simulink model "sampleModel548_pp_1566_1"  (R2021a)
settings: Solver=VariableStepAuto  StartTime=0.0  StopTime=10.0  RelTol=1e-3
undefined symbols (not defined in the file or in its folder): DiscIntNeverNeededParam, Newton, Raphson
libraries: simulink x54, pid_lib x8
(part 1 of 2)
settings Model: Creator=user  LastModifiedBy=user

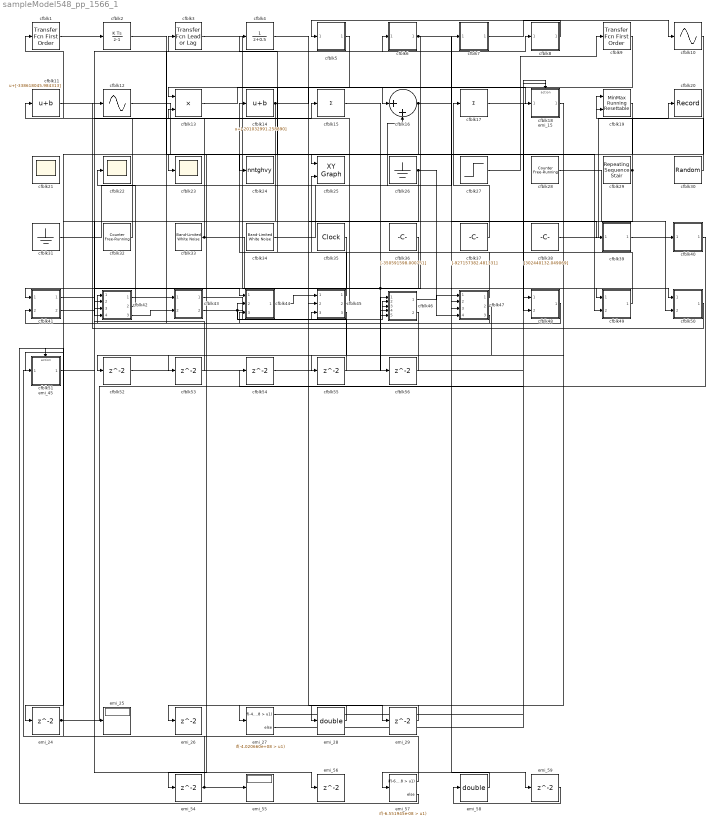
== system sampleModel548_pp_1566_1 ==
  cfblk1 : simulink/Discrete/Transfer Fcn First Order  PoleZ=0.95  ICPrevOutput=0.0  DoSatur=off
  cfblk10 : Sin  TimeSource=Use external signal  SampleTime=0
  cfblk11 : Bias  Bias=[-338618045.984313]
  cfblk12 : Sin  TimeSource=Use external signal  SampleTime=0
  cfblk13 : Product
  cfblk14 : Bias  Bias=[-201032991.258890]
  cfblk15 : Sum  Inputs=+
  cfblk16 : Sum  Inputs=|++
  cfblk17 : Sum  Inputs=+
  cfblk18 : Subsystem  TreatAsAtomicUnit=on
  cfblk19 : simulink/Math Operations/MinMax Running Resettable  Function=min  vinit=0.0
  cfblk2 : DiscreteIntegrator  ICPrevOutput=DiscIntNeverNeededParam  ICPrevScaledInput=DiscIntNeverNeededParam
  cfblk20 : Record  FileSettingsInternal="{\"entries\":[{\"content\":{\"excelSettings\":{\"content\":{},\"type\":\"Streamout.ExcelSettings\"}},\"type\":\"Streamout.FileSettingStorage\",\"uuid\":\"7a93cd99-5695-4368-9288-ae4d8ae2b655\"}],\"packageUris\":[\"http://schema.mathworks.com/mf0/streamout_blocks/R2020a\"],\"version\":\"1.0\"}"  SignalsInternal="{\"entries\":[{\"content\":{\"signals\":[{\"content\":{\"blockPath\":[\"sampleModel548_pp_1566_1/cfblk20\"],\"channel\":[],\"dimensions\":[1],\"domain\":\"samplemodel548_pp_1566_1/cfblk20\",\"lineColor\":\"#b746ff\",\"plots\":[1],\"port\":1,\"sid\":[\"\"],\"signalID\":1494751,\"signalName\":\"cfblk38\"},\"type\":\"RecordBlkView.Signal\",\"uuid\":\"c7f9f908-5acf-44de-b635-a9ae11b3c0ae\"}]},\"type\":\"RecordBlkView.InputSignals\",\"uuid\":\"681cfd0e-31b9-4ca3-9765-5b08f12cf705\"}],\"packageUris\":[\"http://schema.mathworks.com/mf0/streamout_blocks/R2020a\"],\"version\":\"1.0\"}"  VisualizationBindings="{\"sparklinesplugin\":{\"info\":[{\"bindingParametersList\":[],\"subplotID\":1}]}}"
  cfblk21 : Scope
      settings: Floating=on
  cfblk22 : Scope
  cfblk23 : Scope
  cfblk24 : ToWorkspace  VariableName=nntghvy  SaveFormat=Timeseries  SampleTime=-1
  cfblk25 : simulink/Sinks/XY Graph  xmin=-1  xmax=1  ymin=-1  ymax=1  st=-1
  cfblk26 : Ground
  cfblk27 : Step  Time=[40.000000]  Before=[709789414.662240]  After=[776735056.730233]  SampleTime=0
  cfblk28 : simulink/Sources/Counter Free-Running  NumBits=[29.000000]  tsamp=-1
  cfblk29 : simulink/Sources/Repeating Sequence Stair  OutValues=[661742616.793887, -192762915.667570]  tsamp=-1  OutMin=[]  OutMax=[]  OutDataTypeStr=double  OutputDataTypeScalingMode=double  OutDataType=fixdt(0,8)  ConRadixGroup=Best Precision: Vector-wise  OutScaling=2^-12
  cfblk3 : simulink/Discrete/Transfer Fcn Lead or Lag  PoleZ=0.95  ZeroZ=0.75  ICPrevOutput=0.0  ICPrevInput=0.0  DoSatur=off
      settings: SourceProductBaseCode=SL
  cfblk30 : UniformRandomNumber  Minimum=[-3848918818.431031]  Maximum=[6546494102.083925]  Seed=[18894411.000000]  SampleTime=0.1
  cfblk31 : Ground
  cfblk32 : simulink/Sources/Counter Free-Running  NumBits=[47.000000]  tsamp=-1
  cfblk33 : simulink/Sources/Band-Limited White Noise  Cov=[521319541.609249]  Ts=0.1  seed=[6000899315.000000]
  cfblk34 : simulink/Sources/Band-Limited White Noise  Cov=[5907275539.818776]  Ts=0.1  seed=[7621611147.000000]
  cfblk35 : DigitalClock
  cfblk36 : Constant  Value=[-350591598.000751]  SampleTime=1
  cfblk37 : Constant  Value=[-927157382.481331]  SampleTime=1
  cfblk38 : Constant  Value=[302440132.049069]  SampleTime=1
  cfblk39 : Subsystem  TreatAsAtomicUnit=on
  cfblk4 : DiscreteTransferFcn  SampleTime=1
  cfblk40 : Subsystem
  cfblk41 : Subsystem
  cfblk42 : Subsystem
  cfblk43 : Subsystem
  cfblk44 : Subsystem
  cfblk45 : Subsystem
  cfblk46 : Subsystem
  cfblk47 : Subsystem
  cfblk48 : Subsystem
  cfblk49 : Subsystem
  cfblk5 : Subsystem  TreatAsAtomicUnit=on
  cfblk50 : Subsystem
  cfblk51 : Subsystem  TreatAsAtomicUnit=on
  cfblk{52..56} (5 alike) : Delay  SampleTime=1
  cfblk6 : Subsystem  TreatAsAtomicUnit=on
  cfblk7 : Subsystem  TreatAsAtomicUnit=on
  cfblk8 : Subsystem  TreatAsAtomicUnit=on
  cfblk9 : simulink/Discrete/Transfer Fcn First Order  PoleZ=0.95  ICPrevOutput=0.0  DoSatur=off
  emi_15 : Subsystem  TreatAsAtomicUnit=on
  emi_24 : Delay
  emi_25 : Display
  emi_26 : Delay
  emi_27 : If  IfExpression=-4.020660e+08 > u1
  emi_28 : DataTypeConversion  OutDataTypeStr=double
  emi_29 : Delay  InitialCondition=-201032991.2589
  emi_45 : Subsystem  TreatAsAtomicUnit=on
  emi_54 : Delay  SampleTime=1
  emi_55 : Display
  emi_56 : Delay  SampleTime=1
  emi_57 : If  IfExpression=-6.551945e-08 > u1  SampleTime=1
  emi_58 : DataTypeConversion  OutDataTypeStr=double
  emi_59 : Delay  InitialCondition=-3.276e-08
  wires:
  cfblk48/1(cfblk2) -> cfblk42/1(cfblk1)
  cfblk50/1(cfblk2) -> cfblk12/1
  cfblk27/1 -> cfblk9/1
  cfblk3/1 -> cfblk48/2(cfblk11)
  cfblk47/1(cfblk2) -> cfblk14/1
  cfblk9/1 -> cfblk24/1
  cfblk33/1 -> cfblk47/2(cfblk13), cfblk46/5(cfblk16), cfblk11/1
  cfblk13/1 -> cfblk16/1
  cfblk2/1 -> cfblk25/1
  cfblk42/2(cfblk15) -> cfblk22/1
  cfblk1/1 -> cfblk2/1
  cfblk45/1(cfblk2) -> cfblk4/1
  cfblk29/1 -> cfblk19/1, cfblk47/3(cfblk14)
  cfblk36/1 -> cfblk41/1(cfblk1)
  cfblk10/1 -> cfblk23/1
  cfblk31/1 -> cfblk16/2
  cfblk26/1 -> cfblk42/2(cfblk12), cfblk47/4(cfblk15)
  cfblk49/1(cfblk2) -> cfblk25/2
  cfblk41/1(cfblk2) -> cfblk15/1
  cfblk32/1 -> cfblk1/1
  cfblk37/1 -> cfblk17/1
  cfblk30/1 -> cfblk19/2
  cfblk17/1 -> cfblk50/1(cfblk1)
  cfblk28/1 -> cfblk50/2(cfblk7)
  cfblk12/1 -> cfblk49/2(cfblk8)
  cfblk38/1 -> cfblk20/1
  cfblk43/1(cfblk2) -> cfblk46/2(cfblk13)
  cfblk44/1(cfblk2) -> cfblk45/1(cfblk1)
  cfblk43/2(cfblk14) -> cfblk46/3(cfblk14), cfblk45/3(cfblk15)
  cfblk19/1 -> cfblk46/4(cfblk15)
  cfblk41/2(cfblk11) -> cfblk44/1(cfblk1)
  cfblk46/1(cfblk2) -> cfblk47/1(cfblk1)
  cfblk45/2(cfblk16) -> cfblk13/2
  cfblk46/2(cfblk17) -> cfblk41/2(cfblk10)
  cfblk35/1 -> cfblk42/4(cfblk14)
  cfblk42/3(cfblk16) -> cfblk43/2(cfblk13)
  cfblk47/3(cfblk17) -> cfblk44/3(cfblk11)
  cfblk52/1 -> cfblk48/1(cfblk1)
  cfblk47/2(cfblk16) -> cfblk53/1
  cfblk53/1 -> cfblk42/3(cfblk13)
  cfblk40/1(cfblk2) -> cfblk54/1
  cfblk54/1 -> cfblk46/1(cfblk1)
  cfblk45/3(cfblk17) -> cfblk55/1
  cfblk55/1 -> cfblk44/2(cfblk10)
  cfblk15/1 -> cfblk56/1
  cfblk56/1 -> cfblk43/1(cfblk1)
  cfblk4/1 -> cfblk39/1(emi_10)
  cfblk39/1(emi_11) -> cfblk40/1(cfblk1)
  cfblk14/1 -> cfblk18/1(emi_13), emi_24/1, emi_29/1
  cfblk18/1(emi_14) -> cfblk52/1
  emi_24/1 -> emi_15/1(emi_22), emi_25/1
  emi_15/1(emi_23) -> emi_26/1
  emi_27/2 -> cfblk18/Action
  emi_27/1 -> emi_15/Action
  emi_28/1 -> emi_27/1
  emi_29/1 -> emi_28/1
  cfblk5/1(emi_32) -> cfblk13/1
  cfblk11/1 -> cfblk6/1(emi_34)
  cfblk6/1(emi_35) -> cfblk45/2(cfblk14), cfblk49/1(cfblk1)
  cfblk34/1 -> cfblk7/1(emi_37)
  cfblk7/1(emi_38) -> cfblk10/1
  cfblk42/1(cfblk2) -> cfblk8/1(emi_40)
  cfblk8/1(emi_41) -> cfblk5/1(emi_31)
  cfblk16/1 -> cfblk51/1(emi_43), emi_54/1, emi_59/1
  cfblk51/1(emi_44) -> cfblk3/1
  emi_54/1 -> emi_45/1(emi_52), emi_55/1
  emi_45/1(emi_53) -> emi_56/1
  emi_57/2 -> cfblk51/Action
  emi_57/1 -> emi_45/Action
  emi_58/1 -> emi_57/1
  emi_59/1 -> emi_58/1

== system sampleModel548_pp_1566_1/cfblk18 ==
  emi_13 : Inport
  Action Port : ActionPort  ActionPortLabel=else
  cfblk18 : Subsystem  TreatAsAtomicUnit=on
  emi_14 : Outport
  wires:
  emi_13/1 -> cfblk18/1(emi_7)
  cfblk18/1(emi_8) -> emi_14/1

== system sampleModel548_pp_1566_1/cfblk39 ==
  emi_10 : Inport  Partition=on  PartitionDimension=1  PartitionWidth=1  PartitionOffset=0
  For Each : ForEach  DisableCoverage=on
  cfblk39 : Subsystem
  emi_11 : Outport  ConcatenationDimension=1
  wires:
  emi_10/1 -> cfblk39/1(cfblk1)
  cfblk39/1(cfblk2) -> emi_11/1

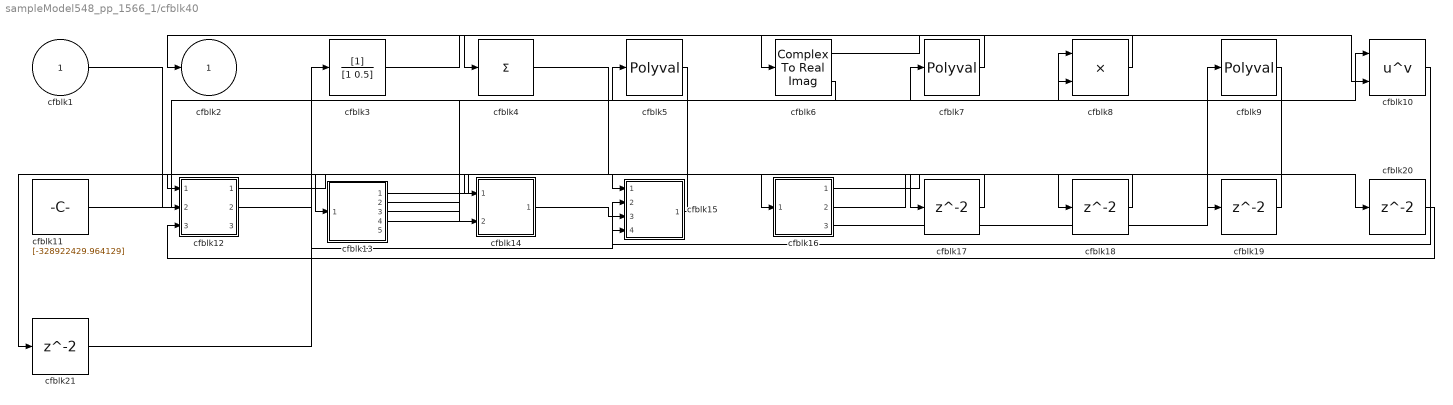
== system sampleModel548_pp_1566_1/cfblk40 ==
  cfblk1 : Inport
  cfblk10 : Math  Operator=pow  SaturateOnIntegerOverflow=on
  cfblk11 : Constant  Value=[-328922429.964129]  SampleTime=1
  cfblk12 : Subsystem
  cfblk13 : Subsystem
  cfblk14 : Subsystem
  cfblk15 : Subsystem
  cfblk16 : Subsystem
  cfblk{17..21} (5 alike) : Delay  SampleTime=1
  cfblk3 : DiscreteFilter  SampleTime=1
  cfblk4 : Sum  Inputs=+
  cfblk5 : Polyval  Coefs=[ +2.081618890e-019, -1.441693666e-014, +4.719686976e-010, -8.536869453e-006, +1.621573104e-001, -8.087801117e+001 ]
  cfblk6 : ComplexToRealImag
  cfblk7 : Polyval  Coefs=[ +2.081618890e-019, -1.441693666e-014, +4.719686976e-010, -8.536869453e-006, +1.621573104e-001, -8.087801117e+001 ]
  cfblk8 : Product
  cfblk9 : Polyval  Coefs=[ +2.081618890e-019, -1.441693666e-014, +4.719686976e-010, -8.536869453e-006, +1.621573104e-001, -8.087801117e+001 ]
  cfblk2 : Outport
  wires:
  cfblk7/1 -> cfblk4/1
  cfblk11/1 -> cfblk10/1
  cfblk3/1 -> cfblk6/1
  cfblk10/1 -> cfblk15/2(cfblk7)
  cfblk6/1 -> cfblk10/2
  cfblk8/1 -> cfblk2/1
  cfblk6/2 -> cfblk5/1
  cfblk12/1(cfblk2) -> cfblk16/1(cfblk1)
  cfblk5/1 -> cfblk12/2(cfblk11)
  cfblk13/2(cfblk14) -> cfblk7/1
  cfblk1/1 -> cfblk14/2(cfblk9)
  cfblk14/1(cfblk2) -> cfblk15/3(cfblk8)
  cfblk16/3(cfblk16) -> cfblk9/1
  cfblk15/1(cfblk2) -> cfblk13/1(cfblk1)
  cfblk13/3(cfblk15) -> cfblk8/1
  cfblk13/4(cfblk16) -> cfblk8/2
  cfblk12/2(cfblk13) -> cfblk15/4(cfblk9)
  cfblk13/1(cfblk2) -> cfblk17/1
  cfblk17/1 -> cfblk14/1(cfblk1)
  cfblk4/1 -> cfblk18/1
  cfblk18/1 -> cfblk15/1(cfblk1)
  cfblk16/1(cfblk2) -> cfblk19/1
  cfblk19/1 -> cfblk12/1(cfblk1)
  cfblk16/2(cfblk15) -> cfblk20/1
  cfblk20/1 -> cfblk12/3(cfblk12)
  cfblk9/1 -> cfblk21/1
  cfblk21/1 -> cfblk3/1

== system sampleModel548_pp_1566_1/cfblk41 ==
  cfblk1 : Inport
  cfblk10 : Inport  Port=2
  cfblk3 : Delay  ShowEnablePort=on  SampleTime=1
      settings: InputPortMap=u0,e6
  cfblk4 : Product  Inputs=*
  cfblk5 : Sqrt  SaturateOnIntegerOverflow=on
  cfblk6 : Sin  TimeSource=Use external signal  SampleTime=0
  cfblk7 : Subsystem
  cfblk8 : Subsystem
  cfblk9 : Subsystem
  cfblk2 : Outport
  cfblk11 : Outport  Port=2
  wires:
  cfblk6/1 -> cfblk2/1
  cfblk3/1 -> cfblk6/1
  cfblk10/1 -> cfblk3/1
  cfblk1/1 -> cfblk7/1(cfblk1)
  cfblk8/1(cfblk2) -> cfblk4/1
  cfblk8/2(cfblk10) -> cfblk5/1
  cfblk5/1 -> cfblk11/1
  cfblk9/1(cfblk2) -> cfblk3/2
  cfblk9/2(cfblk15) -> cfblk8/1(cfblk1)
  cfblk7/1(cfblk2) -> cfblk9/1(cfblk1)
  cfblk7/2(cfblk7) -> cfblk9/2(cfblk13)
  cfblk7/3(cfblk8) -> cfblk9/3(cfblk14)

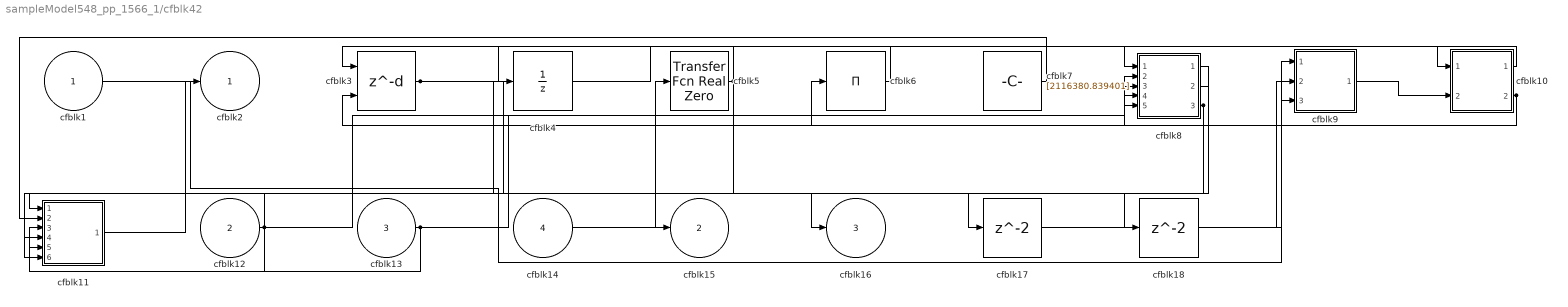
== system sampleModel548_pp_1566_1/cfblk42 ==
  cfblk1 : Inport
  cfblk12 : Inport  Port=2
  cfblk13 : Inport  Port=3
  cfblk14 : Inport  Port=4
  cfblk10 : Subsystem
  cfblk11 : Subsystem
  cfblk17 : Delay  SampleTime=1
  cfblk18 : Delay  SampleTime=1
  cfblk3 : Delay  DelayLengthSource=Input port  SampleTime=1
      settings: InputPortMap=u0,p1
  cfblk4 : UnitDelay  HasFrameUpgradeWarning=on
  cfblk5 : simulink/Discrete/Transfer Fcn Real Zero  ZeroZ=0.75  ICPrevInput=0.0  DoSatur=off
      settings: SourceProductBaseCode=SL
  cfblk6 : Product  Inputs=*
  cfblk7 : Constant  Value=[2116380.839401]  SampleTime=1
  cfblk8 : Subsystem
  cfblk9 : Subsystem
  cfblk2 : Outport
  cfblk15 : Outport  Port=2
  cfblk16 : Outport  Port=3
  wires:
  cfblk3/1 -> cfblk16/1, cfblk18/1
  cfblk6/1 -> cfblk3/1
  cfblk14/1 -> cfblk5/1
  cfblk12/1 -> cfblk11/1(cfblk1), cfblk11/5(cfblk15), cfblk8/4(cfblk13)
  cfblk5/1 -> cfblk4/1, cfblk11/6(cfblk16)
  cfblk7/1 -> cfblk11/2(cfblk12)
  cfblk13/1 -> cfblk11/3(cfblk13), cfblk8/3(cfblk12)
  cfblk1/1 -> cfblk9/1(cfblk1)
  cfblk4/1 -> cfblk10/1(cfblk1)
  cfblk10/1(cfblk2) -> cfblk8/1(cfblk1)
  cfblk9/1(cfblk2) -> cfblk10/2(cfblk16)
  cfblk11/1(cfblk2) -> cfblk2/1
  cfblk10/2(cfblk17) -> cfblk6/1, cfblk8/2(cfblk11), cfblk8/5(cfblk14)
  cfblk8/1(cfblk2) -> cfblk15/1
  cfblk8/3(cfblk16) -> cfblk11/4(cfblk14), cfblk3/2
  cfblk8/2(cfblk15) -> cfblk17/1
  cfblk17/1 -> cfblk9/2(cfblk6)
  cfblk18/1 -> cfblk9/3(cfblk7)

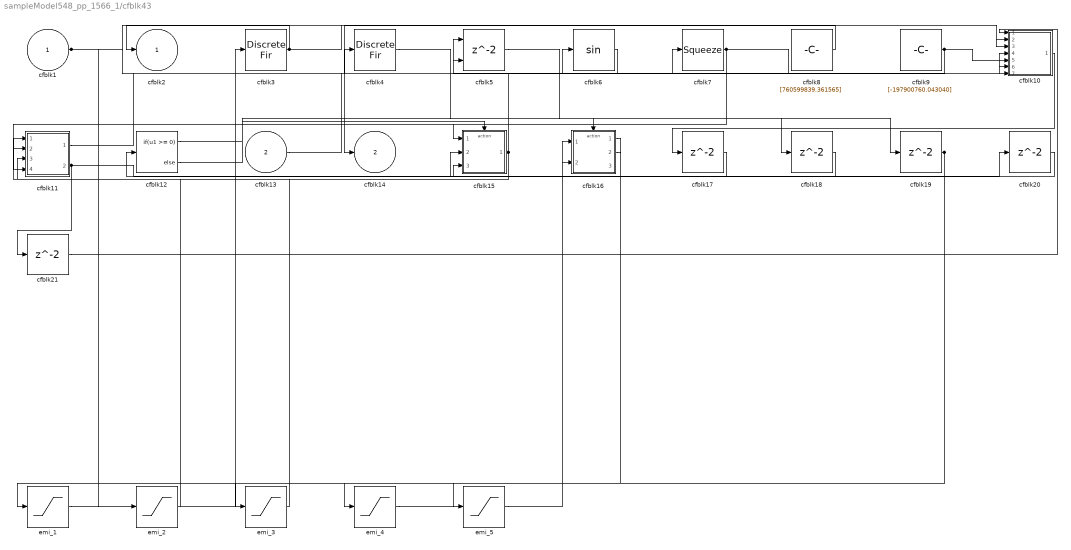
== system sampleModel548_pp_1566_1/cfblk43 ==
  cfblk1 : Inport
  cfblk13 : Inport  Port=2
  cfblk10 : Subsystem
  cfblk11 : Subsystem
  cfblk12 : If  IfExpression=u1 >= 0  SampleTime=1
  cfblk15 : Subsystem  TreatAsAtomicUnit=on
  cfblk16 : Subsystem  TreatAsAtomicUnit=on
  cfblk{17..21} (5 alike) : Delay  SampleTime=1
  cfblk3 : DiscreteFir  SampleTime=1
  cfblk4 : DiscreteFir  SampleTime=1
  cfblk5 : Delay  ShowEnablePort=on  SampleTime=1
      settings: InputPortMap=u0,e6
  cfblk6 : Trigonometry
  cfblk7 : Squeeze
  cfblk8 : Constant  Value=[760599839.361565]  SampleTime=1
  cfblk9 : Constant  Value=[-197900760.043040]  SampleTime=1
  emi_{1..5} (5 alike) : Saturate  UpperLimit=0  LowerLimit=0  ZeroCross=off
  cfblk2 : Outport
  cfblk14 : Outport  Port=2
  wires:
  cfblk15/1(cfblk2) -> cfblk5/1, cfblk11/3(cfblk15)
  cfblk8/1 -> cfblk14/1
  cfblk9/1 -> cfblk6/1, cfblk10/5(cfblk10)
  cfblk11/1(cfblk2) -> cfblk4/1
  cfblk6/1 -> cfblk5/2
  cfblk13/1 -> cfblk7/1
  cfblk11/2(cfblk17) -> cfblk20/1, cfblk21/1
  cfblk3/1 -> cfblk2/1, cfblk10/3(cfblk8)
  cfblk7/1 -> cfblk15/1(cfblk1), cfblk11/4(cfblk16), cfblk10/4(cfblk9), cfblk10/6(cfblk11)
  cfblk1/1 -> cfblk10/2(cfblk7), cfblk10/7(cfblk12), emi_2/1
  cfblk12/1 -> cfblk15/Action
  cfblk12/2 -> cfblk16/Action
  cfblk10/1(cfblk2) -> cfblk17/1
  cfblk17/1 -> cfblk15/2(cfblk10)
  cfblk5/1 -> cfblk18/1
  cfblk18/1 -> cfblk15/3(cfblk11)
  cfblk4/1 -> cfblk19/1
  cfblk20/1 -> cfblk12/1
  cfblk21/1 -> cfblk10/1(cfblk1)
  emi_1/1 -> cfblk3/1
  cfblk19/1 -> emi_1/1, emi_3/1
  emi_2/1 -> cfblk11/1(cfblk1)
  emi_3/1 -> cfblk11/2(cfblk14)
  emi_4/1 -> cfblk16/1(cfblk1)
  cfblk16/1(cfblk2) -> emi_4/1
  emi_5/1 -> cfblk16/2(cfblk9)
  cfblk16/2(cfblk10) -> emi_5/1

== system sampleModel548_pp_1566_1/cfblk44 ==
  cfblk1 : Inport
  cfblk10 : Inport  Port=2
  cfblk11 : Inport  Port=3
  cfblk3 : DiscreteFir  SampleTime=1
  cfblk4 : Delay  ShowEnablePort=on  SampleTime=1
      settings: InputPortMap=u0,e6
  cfblk5 : DiscreteStateSpace
  cfblk6 : Signum
  cfblk7 : Constant  Value=[-388627596.209569]  SampleTime=1
  cfblk8 : Constant  Value=[-19012046.520637]  SampleTime=1
  cfblk9 : Subsystem
  cfblk2 : Outport
  wires:
  cfblk8/1 -> cfblk5/1
  cfblk9/1(cfblk2) -> cfblk4/1
  cfblk1/1 -> cfblk4/2
  cfblk10/1 -> cfblk6/1
  cfblk5/1 -> cfblk3/1
  cfblk7/1 -> cfblk2/1
  cfblk3/1 -> cfblk9/1(cfblk1)
  cfblk6/1 -> cfblk9/2(cfblk11)

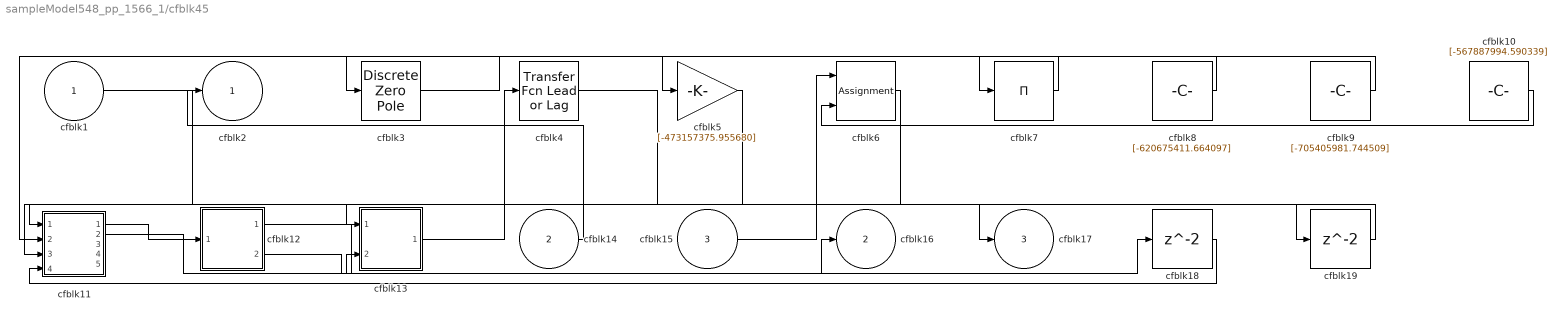
== system sampleModel548_pp_1566_1/cfblk45 ==
  cfblk1 : Inport
  cfblk14 : Inport  Port=2
  cfblk15 : Inport  Port=3
  cfblk10 : Constant  Value=[-567887994.590339]  SampleTime=1
  cfblk11 : Subsystem
  cfblk12 : Subsystem
  cfblk13 : Subsystem
  cfblk18 : Delay  SampleTime=1
  cfblk19 : Delay  SampleTime=1
  cfblk3 : DiscreteZeroPole  Poles=[0 0.5]  Gain=1
  cfblk4 : simulink/Discrete/Transfer Fcn Lead or Lag  PoleZ=0.95  ZeroZ=0.75  ICPrevOutput=0.0  ICPrevInput=0.0  DoSatur=off
      settings: SourceProductBaseCode=SL
  cfblk5 : Gain  Gain=[-473157375.955680]
  cfblk6 : Assignment  DiagnosticForDimensions=Warning  IndexOptions=Index vector (dialog)  Indices=1  OutputSizes=1
  cfblk7 : Product  Inputs=*
  cfblk8 : Constant  Value=[-620675411.664097]  SampleTime=1
  cfblk9 : Constant  Value=[-705405981.744509]  SampleTime=1
  cfblk2 : Outport
  cfblk16 : Outport  Port=2
  cfblk17 : Outport  Port=3
  wires:
  cfblk5/1 -> cfblk11/1(cfblk1)
  cfblk7/1 -> cfblk11/2(cfblk9)
  cfblk12/1(cfblk2) -> cfblk16/1
  cfblk1/1 -> cfblk17/1
  cfblk13/1(cfblk2) -> cfblk4/1
  cfblk3/1 -> cfblk7/1
  cfblk15/1 -> cfblk6/1
  cfblk9/1 -> cfblk3/1
  cfblk6/1 -> cfblk11/3(cfblk10)
  cfblk8/1 -> cfblk5/1
  cfblk11/1(cfblk2) -> cfblk12/1(cfblk1)
  cfblk10/1 -> cfblk6/2
  cfblk14/1 -> cfblk2/1
  cfblk11/2(cfblk12) -> cfblk13/2(cfblk9)
  cfblk12/2(cfblk10) -> cfblk18/1
  cfblk18/1 -> cfblk11/4(cfblk11)
  cfblk4/1 -> cfblk19/1
  cfblk19/1 -> cfblk13/1(cfblk1)

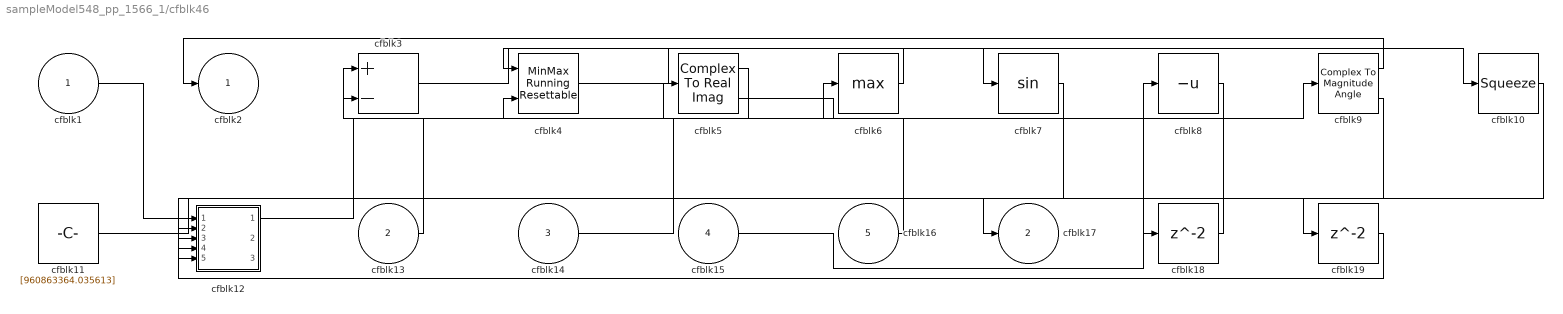
== system sampleModel548_pp_1566_1/cfblk46 ==
  cfblk1 : Inport
  cfblk13 : Inport  Port=2
  cfblk14 : Inport  Port=3
  cfblk15 : Inport  Port=4
  cfblk16 : Inport  Port=5
  cfblk10 : Squeeze
  cfblk11 : Constant  Value=[960863364.035613]  SampleTime=1
  cfblk12 : Subsystem
  cfblk18 : Delay  SampleTime=1
  cfblk19 : Delay  SampleTime=1
  cfblk3 : Sum  Inputs=+-
  cfblk4 : simulink/Math Operations/MinMax Running Resettable  Function=min  vinit=0.0
  cfblk5 : ComplexToRealImag
  cfblk6 : MinMax  Function=max
  cfblk7 : Trigonometry
  cfblk8 : UnaryMinus
  cfblk9 : ComplexToMagnitudeAngle
  cfblk2 : Outport
  cfblk17 : Outport  Port=2
  wires:
  cfblk3/1 -> cfblk7/1
  cfblk11/1 -> cfblk17/1
  cfblk9/1 -> cfblk2/1
  cfblk1/1 -> cfblk12/1(cfblk1)
  cfblk6/1 -> cfblk4/1
  cfblk13/1 -> cfblk3/1
  cfblk5/1 -> cfblk4/2
  cfblk4/1 -> cfblk10/1
  cfblk15/1 -> cfblk8/1
  cfblk7/1 -> cfblk12/2(cfblk11)
  cfblk16/1 -> cfblk3/2
  cfblk12/1(cfblk2) -> cfblk5/1
  cfblk5/2 -> cfblk9/1
  cfblk14/1 -> cfblk6/1
  cfblk8/1 -> cfblk12/5(cfblk14)
  cfblk10/1 -> cfblk18/1
  cfblk18/1 -> cfblk12/3(cfblk12)
  cfblk9/2 -> cfblk19/1
  cfblk19/1 -> cfblk12/4(cfblk13)

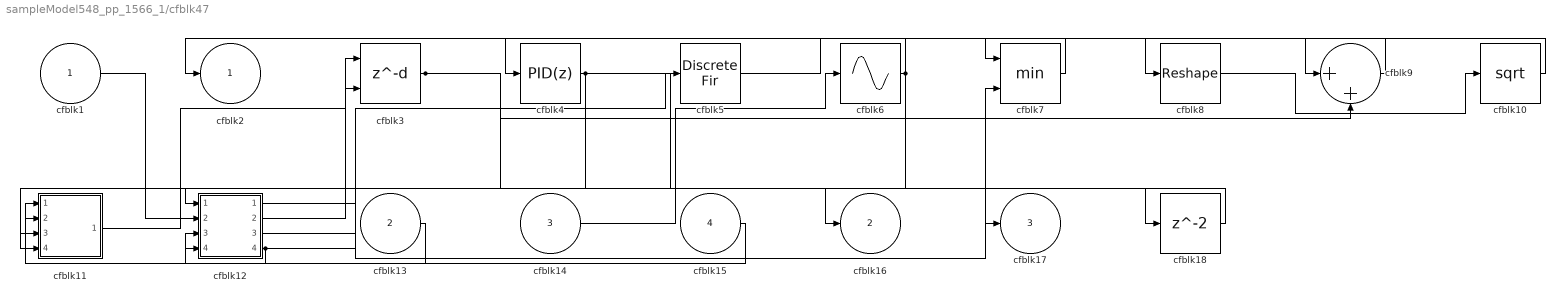
== system sampleModel548_pp_1566_1/cfblk47 ==
  cfblk1 : Inport
  cfblk13 : Inport  Port=2
  cfblk14 : Inport  Port=3
  cfblk15 : Inport  Port=4
  cfblk10 : Sqrt  SaturateOnIntegerOverflow=on
  cfblk11 : Subsystem
  cfblk12 : Subsystem
  cfblk18 : Delay  SampleTime=1
  cfblk3 : Delay  DelayLengthSource=Input port  SampleTime=1
      settings: InputPortMap=u0,p1
  cfblk4 : pid_lib/PID Controller  Controller=PID  Form=Parallel  TimeDomain=Discrete-time  UseExternalTs=off  SampleTime=1  IntegratorMethod=Forward Euler  FilterMethod=Forward Euler  ControllerParametersSource=internal  P=1  I=1  D=0  UseFilter=on  N=100  TunerSelectOption=Transfer Function Based (PID Tuner App)  InitialConditionSource=internal  InitialConditionForIntegrator=0  InitialConditionForFilter=0  DifferentiatorICPrevScaledInput=0  ExternalReset=none  TrackingMode=off  Kt=1  LimitOutput=off  SatLimitsSource=internal  UpperSaturationLimit=inf  LowerSaturationLimit=-inf  LinearizeAsGain=off  AntiWindupMode=none  Kb=1  POutMin=[]  POutMax=[]  IOutMin=[]  IOutMax=[]  DOutMin=[]  DOutMax=[]  NOutMin=[]  NOutMax=[]  SumOutMin=[]  SumOutMax=[]  SaturationOutMin=[]  SaturationOutMax=[]  PParamMin=[]  PParamMax=[]  IParamMin=[]  IParamMax=[]  DParamMin=[]  DParamMax=[]  NParamMin=[]  NParamMax=[]  KbParamMin=[]  KbParamMax=[]  KtParamMin=[]  KtParamMax=[]  KbOutMin=[]  KbOutMax=[]  KtOutMin=[]  KtOutMax=[]  IntegratorOutMin=[]  IntegratorOutMax=[]  FilterOutMin=[]  FilterOutMax=[]  SumI1OutMin=[]  SumI1OutMax=[]  SumI2OutMin=[]  SumI2OutMax=[]  SumI3OutMin=[]  SumI3OutMax=[]  SumI4OutMin=[]  SumI4OutMax=[]  SumDOutMin=[]  SumDOutMax=[]  DifferentiatorOutMin=[]  DifferentiatorOutMax=[]  FilterDiffOutCoefMin=[]  FilterDiffOutCoefMax=[]  ReciprocalOutMin=[]  ReciprocalOutMax=[]  SumDenOutMin=[]  SumDenOutMax=[]  SumNumOutMin=[]  SumNumOutMax=[]  DivideOutMin=[]  DivideOutMax=[]  UdiffTsProdOutMin=[]  UdiffTsProdOutMax=[]  NTsProdOutMin=[]  NTsProdOutMax=[]  UintegralTsProdOutMin=[]  UintegralTsProdOutMax=[]  UngainTsProdOutMin=[]  UngainTsProdOutMax=[]  IntegratorContinuousStateAttributes=''  IntegratorStateMustResolveToSignalObject=off  IntegratorRTWStateStorageClass=Auto  FilterContinuousStateAttributes=''  FilterStateMustResolveToSignalObject=off  FilterRTWStateStorageClass=Auto  ParallelPVariant=InternalParameters  IdealPVariant=Disabled  IVariant=InternalParameters  DVariant=InternalParameters  IntegratorVariant=Discrete  SatVariant=Disabled  AWVariant=Passthrough  PCopyVariant=Disabled  TRVariant=Disabled  FdbkBlocksVariant=Forward  IdealPFdbkVariant=Disabled  SatFdbkVariant=Disabled  DerivativeFilterVariant=ForwardEulerFilter  NVariant=InternalParameters  NCopyVariant=Disabled  FilterICVariant=InternalICsFilter  IntegratorICVariant=InternalICs  ExternalResetVariant=Disabled  TRSumVariant=Passthrough  SumFdbkVariant=Disabled  SumVariant=Sum_PID  TsampFilterVariant=InternalTs  TsampNgainVariant=Passthrough  TsampIntegralVariant=Passthrough  ExternalSaturationOutDataTypeStr=Inherit: Same as second input
  cfblk5 : DiscreteFir  SampleTime=1
  cfblk6 : Sin  TimeSource=Use external signal  SampleTime=0
  cfblk7 : MinMax  Inputs=2
  cfblk8 : Reshape
  cfblk9 : Sum  Inputs=|++
  cfblk2 : Outport
  cfblk16 : Outport  Port=2
  cfblk17 : Outport  Port=3
  wires:
  cfblk4/1 -> cfblk16/1, cfblk11/4(cfblk9)
  cfblk14/1 -> cfblk6/1
  cfblk10/1 -> cfblk7/1
  cfblk6/1 -> cfblk4/1, cfblk11/3(cfblk8)
  cfblk3/1 -> cfblk9/2, cfblk18/1
  cfblk1/1 -> cfblk12/2(cfblk10)
  cfblk12/1(cfblk2) -> cfblk7/2
  cfblk5/1 -> cfblk9/1
  cfblk13/1 -> cfblk12/3(cfblk11)
  cfblk8/1 -> cfblk10/1
  cfblk12/2(cfblk13) -> cfblk3/1
  cfblk7/1 -> cfblk2/1
  cfblk9/1 -> cfblk8/1
  cfblk12/3(cfblk14) -> cfblk17/1
  cfblk11/1(cfblk2) -> cfblk3/2
  cfblk15/1 -> cfblk12/4(cfblk12)
  cfblk12/4(cfblk15) -> cfblk5/1, cfblk11/1(cfblk1), cfblk11/2(cfblk7)
  cfblk18/1 -> cfblk12/1(cfblk1)

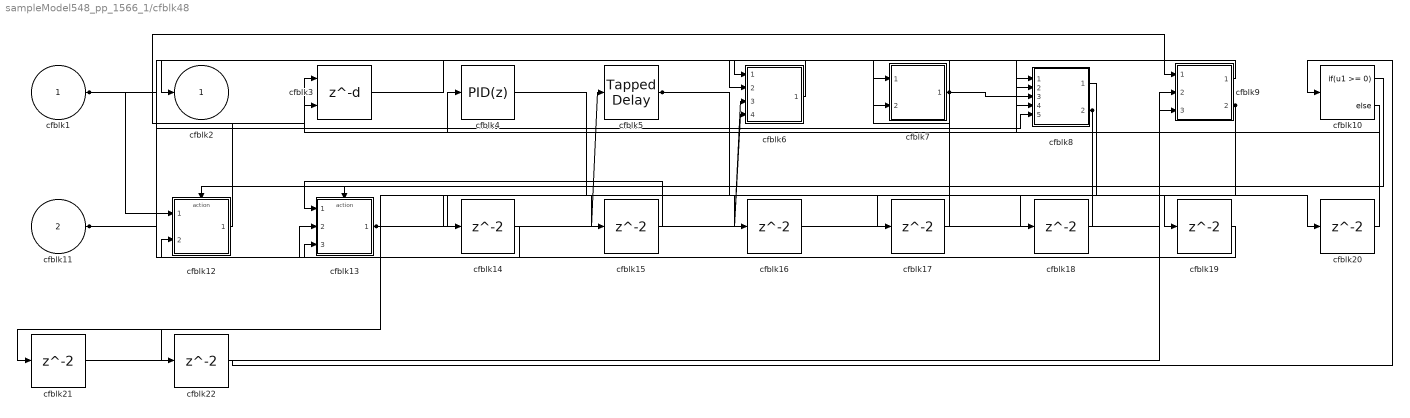
== system sampleModel548_pp_1566_1/cfblk48 ==
  cfblk1 : Inport
  cfblk11 : Inport  Port=2
  cfblk10 : If  IfExpression=u1 >= 0  SampleTime=1
  cfblk12 : Subsystem  TreatAsAtomicUnit=on
  cfblk13 : Subsystem  TreatAsAtomicUnit=on
  cfblk{14..22} (9 alike) : Delay  SampleTime=1
  cfblk3 : Delay  DelayLengthSource=Input port  SampleTime=1
      settings: InputPortMap=u0,p1
  cfblk4 : pid_lib/PID Controller  Controller=PID  Form=Parallel  TimeDomain=Discrete-time  UseExternalTs=off  SampleTime=1  IntegratorMethod=Forward Euler  FilterMethod=Forward Euler  ControllerParametersSource=internal  P=1  I=1  D=0  UseFilter=on  N=100  TunerSelectOption=Transfer Function Based (PID Tuner App)  InitialConditionSource=internal  InitialConditionForIntegrator=0  InitialConditionForFilter=0  DifferentiatorICPrevScaledInput=0  ExternalReset=none  TrackingMode=off  Kt=1  LimitOutput=off  SatLimitsSource=internal  UpperSaturationLimit=inf  LowerSaturationLimit=-inf  LinearizeAsGain=off  AntiWindupMode=none  Kb=1  POutMin=[]  POutMax=[]  IOutMin=[]  IOutMax=[]  DOutMin=[]  DOutMax=[]  NOutMin=[]  NOutMax=[]  SumOutMin=[]  SumOutMax=[]  SaturationOutMin=[]  SaturationOutMax=[]  PParamMin=[]  PParamMax=[]  IParamMin=[]  IParamMax=[]  DParamMin=[]  DParamMax=[]  NParamMin=[]  NParamMax=[]  KbParamMin=[]  KbParamMax=[]  KtParamMin=[]  KtParamMax=[]  KbOutMin=[]  KbOutMax=[]  KtOutMin=[]  KtOutMax=[]  IntegratorOutMin=[]  IntegratorOutMax=[]  FilterOutMin=[]  FilterOutMax=[]  SumI1OutMin=[]  SumI1OutMax=[]  SumI2OutMin=[]  SumI2OutMax=[]  SumI3OutMin=[]  SumI3OutMax=[]  SumI4OutMin=[]  SumI4OutMax=[]  SumDOutMin=[]  SumDOutMax=[]  DifferentiatorOutMin=[]  DifferentiatorOutMax=[]  FilterDiffOutCoefMin=[]  FilterDiffOutCoefMax=[]  ReciprocalOutMin=[]  ReciprocalOutMax=[]  SumDenOutMin=[]  SumDenOutMax=[]  SumNumOutMin=[]  SumNumOutMax=[]  DivideOutMin=[]  DivideOutMax=[]  UdiffTsProdOutMin=[]  UdiffTsProdOutMax=[]  NTsProdOutMin=[]  NTsProdOutMax=[]  UintegralTsProdOutMin=[]  UintegralTsProdOutMax=[]  UngainTsProdOutMin=[]  UngainTsProdOutMax=[]  IntegratorContinuousStateAttributes=''  IntegratorStateMustResolveToSignalObject=off  IntegratorRTWStateStorageClass=Auto  FilterContinuousStateAttributes=''  FilterStateMustResolveToSignalObject=off  FilterRTWStateStorageClass=Auto  ParallelPVariant=InternalParameters  IdealPVariant=Disabled  IVariant=InternalParameters  DVariant=InternalParameters  IntegratorVariant=Discrete  SatVariant=Disabled  AWVariant=Passthrough  PCopyVariant=Disabled  TRVariant=Disabled  FdbkBlocksVariant=Forward  IdealPFdbkVariant=Disabled  SatFdbkVariant=Disabled  DerivativeFilterVariant=ForwardEulerFilter  NVariant=InternalParameters  NCopyVariant=Disabled  FilterICVariant=InternalICsFilter  IntegratorICVariant=InternalICs  ExternalResetVariant=Disabled  TRSumVariant=Passthrough  SumFdbkVariant=Disabled  SumVariant=Sum_PID  TsampFilterVariant=InternalTs  TsampNgainVariant=Passthrough  TsampIntegralVariant=Passthrough  ExternalSaturationOutDataTypeStr=Inherit: Same as second input
  cfblk5 : simulink/Discrete/Tapped Delay  vinit=0.0  samptime=-1  NumDelays=1  DelayOrder=Oldest  includeCurrent=off
  cfblk6 : Subsystem
  cfblk7 : Subsystem
  cfblk8 : Subsystem
  cfblk9 : Subsystem
  cfblk2 : Outport
  wires:
  cfblk5/1 -> cfblk17/1, cfblk18/1, cfblk19/1
  cfblk1/1 -> cfblk12/1(cfblk1), cfblk6/2(cfblk11), cfblk8/5(cfblk13)
  cfblk7/1(cfblk2) -> cfblk6/1(cfblk1), cfblk8/3(cfblk11), cfblk14/1
  cfblk6/1(cfblk2) -> cfblk2/1
  cfblk12/1(cfblk2) -> cfblk9/1(cfblk1)
  cfblk8/2(cfblk14) -> cfblk4/1, cfblk21/1
  cfblk3/1 -> cfblk8/2(cfblk10)
  cfblk9/1(cfblk2) -> cfblk7/2(cfblk8)
  cfblk11/1 -> cfblk3/1, cfblk13/3(cfblk13)
  cfblk9/2(cfblk14) -> cfblk3/2, cfblk22/1
  cfblk13/1(cfblk2) -> cfblk5/1, cfblk6/3(cfblk12), cfblk6/4(cfblk13), cfblk16/1
  cfblk10/1 -> cfblk12/Action
  cfblk10/2 -> cfblk13/Action
  cfblk14/1 -> cfblk12/2(cfblk10)
  cfblk8/1(cfblk2) -> cfblk15/1
  cfblk15/1 -> cfblk13/1(cfblk1)
  cfblk16/1 -> cfblk9/2(cfblk12)
  cfblk17/1 -> cfblk7/1(cfblk1)
  cfblk18/1 -> cfblk8/4(cfblk12)
  cfblk19/1 -> cfblk13/2(cfblk12)
  cfblk4/1 -> cfblk20/1
  cfblk20/1 -> cfblk8/1(cfblk1)
  cfblk21/1 -> cfblk9/3(cfblk13)
  cfblk22/1 -> cfblk10/1

== system sampleModel548_pp_1566_1/cfblk49 ==
  cfblk1 : Inport
  cfblk8 : Inport  Port=2
  cfblk{3,9..11} (4 alike) : Delay  SampleTime=1
  cfblk4 : ComplexToRealImag
  cfblk5 : Reshape
  cfblk6 : Math  Operator=pow  SaturateOnIntegerOverflow=on
  cfblk7 : Subsystem
  cfblk2 : Outport
  wires:
  cfblk1/1 -> cfblk2/1
  cfblk8/1 -> cfblk6/1
  cfblk3/1 -> cfblk7/2(cfblk13)
  cfblk4/1 -> cfblk7/3(cfblk14)
  cfblk4/2 -> cfblk5/1
  cfblk7/1(cfblk2) -> cfblk6/2
  cfblk6/1 -> cfblk9/1
  cfblk9/1 -> cfblk7/1(cfblk1)
  cfblk7/2(cfblk15) -> cfblk10/1
  cfblk10/1 -> cfblk3/1
  cfblk5/1 -> cfblk11/1
  cfblk11/1 -> cfblk4/1

== system sampleModel548_pp_1566_1/cfblk5 ==
  emi_31 : Inport  Partition=on  PartitionDimension=1  PartitionWidth=1  PartitionOffset=0
  For Each : ForEach  DisableCoverage=on
  cfblk5 : DiscreteTransferFcn  SampleTime=1
  emi_32 : Outport  ConcatenationDimension=1
  wires:
  emi_31/1 -> cfblk5/1
  cfblk5/1 -> emi_32/1

== system sampleModel548_pp_1566_1/cfblk50 ==
  cfblk1 : Inport
  cfblk7 : Inport  Port=2
  cfblk3 : DiscreteZeroPole  Poles=[0 0.5]  Gain=1
  cfblk4 : MinMax  Function=max
  cfblk5 : Rounding
  cfblk6 : Subsystem
  cfblk8 : Delay  SampleTime=1
  cfblk9 : Delay  SampleTime=1
  cfblk2 : Outport
  wires:
  cfblk7/1 -> cfblk4/1
  cfblk6/1(cfblk2) -> cfblk2/1
  cfblk1/1 -> cfblk6/1(cfblk1)
  cfblk4/1 -> cfblk6/2(cfblk12)
  cfblk5/1 -> cfblk3/1
  cfblk6/2(cfblk15) -> cfblk5/1
  cfblk3/1 -> cfblk8/1, cfblk9/1
  cfblk8/1 -> cfblk6/3(cfblk13)
  cfblk9/1 -> cfblk6/4(cfblk14)

== system sampleModel548_pp_1566_1/cfblk51 ==
  emi_43 : Inport
  Action Port : ActionPort  ActionPortLabel=else
  cfblk51 : Delay  SampleTime=1
  emi_44 : Outport
  wires:
  emi_43/1 -> cfblk51/1
  cfblk51/1 -> emi_44/1

== system sampleModel548_pp_1566_1/cfblk6 ==
  emi_34 : Inport  Partition=on  PartitionDimension=1  PartitionWidth=1  PartitionOffset=0
  For Each : ForEach  DisableCoverage=on
  cfblk6 : DiscreteFir  SampleTime=1
  emi_35 : Outport  ConcatenationDimension=1
  wires:
  emi_34/1 -> cfblk6/1
  cfblk6/1 -> emi_35/1

== system sampleModel548_pp_1566_1/cfblk7 ==
  emi_37 : Inport  Partition=on  PartitionDimension=1  PartitionWidth=1  PartitionOffset=0
  For Each : ForEach  DisableCoverage=on
  cfblk7 : DiscreteFir  SampleTime=1
  emi_38 : Outport  ConcatenationDimension=1
  wires:
  emi_37/1 -> cfblk7/1
  cfblk7/1 -> emi_38/1

== system sampleModel548_pp_1566_1/cfblk8 ==
  emi_40 : Inport  Partition=on  PartitionDimension=1  PartitionWidth=1  PartitionOffset=0
  For Each : ForEach  DisableCoverage=on
  cfblk8 : simulink/Discrete/Tapped Delay  vinit=0.0  samptime=-1  NumDelays=1  DelayOrder=Oldest  includeCurrent=off
  emi_41 : Outport  ConcatenationDimension=1
  wires:
  emi_40/1 -> cfblk8/1
  cfblk8/1 -> emi_41/1

== system sampleModel548_pp_1566_1/emi_15 ==
  emi_22 : Inport
  Action Port : ActionPort  ActionPortLabel=if(-4.020660e+08 > u1)
  emi_19 : Trigonometry
  emi_20 : MinMax
  emi_21 : Trigonometry
  emi_23 : Outport
  wires:
  emi_22/1 -> emi_19/1
  emi_19/1 -> emi_20/1
  emi_20/1 -> emi_21/1

== system sampleModel548_pp_1566_1/emi_45 ==
  emi_52 : Inport
  Action Port : ActionPort  ActionPortLabel=if(-6.551945e-08 > u1)
  emi_49 : Gain  SampleTime=1
  emi_50 : Math  SampleTime=1  SaturateOnIntegerOverflow=on
  emi_51 : Gain  SampleTime=1
  emi_53 : Outport
  wires:
  emi_52/1 -> emi_49/1
  emi_49/1 -> emi_50/1
  emi_50/1 -> emi_51/1

== system sampleModel548_pp_1566_1/cfblk18/cfblk18 ==
  emi_7 : Inport  Partition=on  PartitionDimension=1  PartitionWidth=1  PartitionOffset=0
  For Each : ForEach  DisableCoverage=on
  cfblk18 : Sqrt  Operator=rSqrt  AlgorithmType=Newton-Raphson  SaturateOnIntegerOverflow=on
  emi_8 : Outport  ConcatenationDimension=1
  wires:
  cfblk18/1 -> emi_8/1
  emi_7/1 -> cfblk18/1

== system sampleModel548_pp_1566_1/cfblk39/cfblk39 ==
  cfblk1 : Inport
  cfblk10 : Subsystem
  cfblk11 : Subsystem
  cfblk12 : Subsystem
  cfblk{3,13..17} (6 alike) : Delay  SampleTime=1
  cfblk4 : Product
  cfblk5 : Constant  Value=[642194864.641767]  SampleTime=1
  cfblk6 : Subsystem
  cfblk7 : Subsystem
  cfblk8 : Subsystem
  cfblk9 : Subsystem
  cfblk2 : Outport
  wires:
  cfblk17/1 -> cfblk10/2(cfblk13)
  cfblk16/1 -> cfblk9/2(cfblk9)
  cfblk15/1 -> cfblk4/2
  cfblk14/1 -> cfblk9/1(cfblk1)
  cfblk13/1 -> cfblk6/1(cfblk1)
  cfblk6/2(cfblk10) -> cfblk11/2(cfblk12), cfblk7/3(cfblk14), cfblk10/3(cfblk14)
  cfblk10/3(cfblk16) -> cfblk8/1(cfblk1)
  cfblk10/2(cfblk15) -> cfblk4/1
  cfblk10/1(cfblk2) -> cfblk12/2(cfblk7)
  cfblk9/2(cfblk11) -> cfblk17/1, cfblk8/2(cfblk6)
  cfblk12/1(cfblk2) -> cfblk2/1
  cfblk1/1 -> cfblk6/2(cfblk9)
  cfblk3/1 -> cfblk11/1(cfblk1)
  cfblk4/1 -> cfblk13/1, cfblk9/3(cfblk10)
  cfblk11/1(cfblk2) -> cfblk10/1(cfblk1)
  cfblk6/1(cfblk2) -> cfblk3/1
  cfblk7/1(cfblk2) -> cfblk16/1, cfblk15/1, cfblk14/1
  cfblk9/1(cfblk2) -> cfblk7/2(cfblk13)
  cfblk8/1(cfblk2) -> cfblk7/1(cfblk1)
  cfblk5/1 -> cfblk8/3(cfblk7), cfblk7/4(cfblk15), cfblk12/1(cfblk1)

== system sampleModel548_pp_1566_1/cfblk40/cfblk12 ==
  cfblk1 : Inport
  cfblk11 : Inport  Port=2
  cfblk12 : Inport  Port=3
  cfblk10 : Constant  Value=[461016352.105140]  SampleTime=1
  cfblk3 : DiscreteTransferFcn  SampleTime=1
  cfblk4 : simulink/Discrete/Tapped Delay  vinit=0.0  samptime=-1  NumDelays=1  DelayOrder=Oldest  includeCurrent=off
  cfblk5 : MinMax  Inputs=2
  cfblk6 : Abs
  cfblk7 : Trigonometry
  cfblk8 : Sum  Inputs=|++
  cfblk9 : Constant  Value=[-205464524.768609]  SampleTime=1
  cfblk2 : Outport
  cfblk13 : Outport  Port=2
  cfblk14 : Outport  Port=3
  wires:
  cfblk7/1 -> cfblk4/1
  cfblk10/1 -> cfblk3/1
  cfblk11/1 -> cfblk8/1
  cfblk12/1 -> cfblk2/1
  cfblk3/1 -> cfblk5/1
  cfblk4/1 -> cfblk8/2
  cfblk5/1 -> cfblk6/1
  cfblk6/1 -> cfblk13/1
  cfblk1/1 -> cfblk14/1
  cfblk8/1 -> cfblk5/2
  cfblk9/1 -> cfblk7/1

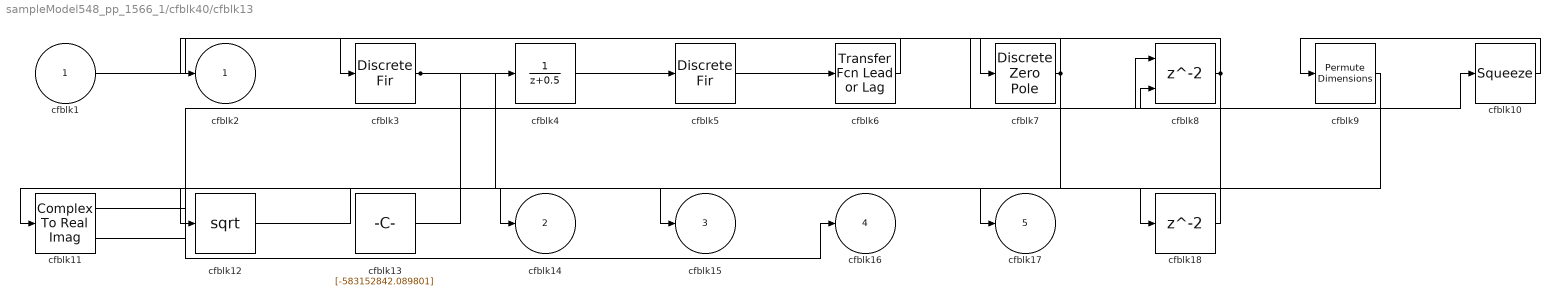
== system sampleModel548_pp_1566_1/cfblk40/cfblk13 ==
  cfblk1 : Inport
  cfblk10 : Squeeze
  cfblk11 : ComplexToRealImag
  cfblk12 : Sqrt  SaturateOnIntegerOverflow=on
  cfblk13 : Constant  Value=[-583152842.089801]  SampleTime=1
  cfblk18 : Delay  SampleTime=1
  cfblk3 : DiscreteFir  SampleTime=1
  cfblk4 : DiscreteTransferFcn  SampleTime=1
  cfblk5 : DiscreteFir  SampleTime=1
  cfblk6 : simulink/Discrete/Transfer Fcn Lead or Lag  PoleZ=0.95  ZeroZ=0.75  ICPrevOutput=0.0  ICPrevInput=0.0  DoSatur=off
      settings: SourceProductBaseCode=SL
  cfblk7 : DiscreteZeroPole  Poles=[0 0.5]  Gain=1
  cfblk8 : Delay  ShowEnablePort=on  SampleTime=1
      settings: InputPortMap=u0,e6
  cfblk9 : PermuteDimensions
  cfblk2 : Outport
  cfblk14 : Outport  Port=2
  cfblk15 : Outport  Port=3
  cfblk16 : Outport  Port=4
  cfblk17 : Outport  Port=5
  wires:
  cfblk8/1 -> cfblk7/1, cfblk14/1
  cfblk10/1 -> cfblk9/1
  cfblk13/1 -> cfblk4/1
  cfblk1/1 -> cfblk10/1
  cfblk4/1 -> cfblk5/1
  cfblk6/1 -> cfblk2/1
  cfblk7/1 -> cfblk3/1, cfblk12/1
  cfblk3/1 -> cfblk15/1, cfblk18/1
  cfblk5/1 -> cfblk6/1
  cfblk11/1 -> cfblk16/1
  cfblk12/1 -> cfblk17/1
  cfblk9/1 -> cfblk11/1
  cfblk11/2 -> cfblk8/2
  cfblk18/1 -> cfblk8/1

== system sampleModel548_pp_1566_1/cfblk40/cfblk14 ==
  cfblk1 : Inport
  cfblk9 : Inport  Port=2
  cfblk10 : Delay  SampleTime=1
  cfblk3 : DiscreteZeroPole  Poles=[0 0.5]  Gain=1
  cfblk4 : DiscreteTransferFcn  SampleTime=1
  cfblk5 : DiscreteStateSpace
  cfblk6 : Product  Inputs=**
  cfblk7 : DotProduct  InputSameDT=on  OutDataTypeStr=Inherit: Inherit via internal rule
  cfblk8 : Product  Inputs=*
  cfblk2 : Outport
  wires:
  cfblk8/1 -> cfblk5/1
  cfblk5/1 -> cfblk3/1
  cfblk7/1 -> cfblk6/1
  cfblk1/1 -> cfblk8/1
  cfblk3/1 -> cfblk7/2, cfblk2/1
  cfblk9/1 -> cfblk6/2
  cfblk6/1 -> cfblk4/1
  cfblk4/1 -> cfblk10/1
  cfblk10/1 -> cfblk7/1

== system sampleModel548_pp_1566_1/cfblk40/cfblk15 ==
  cfblk1 : Inport
  cfblk7 : Inport  Port=2
  cfblk8 : Inport  Port=3
  cfblk9 : Inport  Port=4
  cfblk3 : simulink/Discrete/Transfer Fcn Real Zero  ZeroZ=0.75  ICPrevInput=0.0  DoSatur=off
      settings: SourceProductBaseCode=SL
  cfblk4 : Trigonometry
  cfblk5 : Sqrt  SaturateOnIntegerOverflow=on
  cfblk6 : Math  Operator=transpose  SaturateOnIntegerOverflow=on
  cfblk2 : Outport
  wires:
  cfblk8/1 -> cfblk4/1
  cfblk6/1 -> cfblk5/1
  cfblk3/1 -> cfblk2/1
  cfblk7/1 -> cfblk6/1
  cfblk5/1 -> cfblk3/1

== system sampleModel548_pp_1566_1/cfblk40/cfblk16 ==
  cfblk1 : Inport
  cfblk10 : Polyval  Coefs=[ +2.081618890e-019, -1.441693666e-014, +4.719686976e-010, -8.536869453e-006, +1.621573104e-001, -8.087801117e+001 ]
  cfblk11 : Sum  Inputs=+-
  cfblk12 : Constant  Value=[948608542.431954]  SampleTime=1
  cfblk13 : Constant  Value=[-616578977.498144]  SampleTime=1
  cfblk14 : Constant  Value=[-310376577.440850]  SampleTime=1
  cfblk3 : Delay  DelayLengthSource=Input port  SampleTime=1
      settings: InputPortMap=u0,p1
  cfblk4 : pid_lib/PID Controller  Controller=PID  Form=Parallel  TimeDomain=Discrete-time  UseExternalTs=off  SampleTime=1  IntegratorMethod=Forward Euler  FilterMethod=Forward Euler  ControllerParametersSource=internal  P=1  I=1  D=0  UseFilter=on  N=100  TunerSelectOption=Transfer Function Based (PID Tuner App)  InitialConditionSource=internal  InitialConditionForIntegrator=0  InitialConditionForFilter=0  DifferentiatorICPrevScaledInput=0  ExternalReset=none  TrackingMode=off  Kt=1  LimitOutput=off  SatLimitsSource=internal  UpperSaturationLimit=inf  LowerSaturationLimit=-inf  LinearizeAsGain=off  AntiWindupMode=none  Kb=1  POutMin=[]  POutMax=[]  IOutMin=[]  IOutMax=[]  DOutMin=[]  DOutMax=[]  NOutMin=[]  NOutMax=[]  SumOutMin=[]  SumOutMax=[]  SaturationOutMin=[]  SaturationOutMax=[]  PParamMin=[]  PParamMax=[]  IParamMin=[]  IParamMax=[]  DParamMin=[]  DParamMax=[]  NParamMin=[]  NParamMax=[]  KbParamMin=[]  KbParamMax=[]  KtParamMin=[]  KtParamMax=[]  KbOutMin=[]  KbOutMax=[]  KtOutMin=[]  KtOutMax=[]  IntegratorOutMin=[]  IntegratorOutMax=[]  FilterOutMin=[]  FilterOutMax=[]  SumI1OutMin=[]  SumI1OutMax=[]  SumI2OutMin=[]  SumI2OutMax=[]  SumI3OutMin=[]  SumI3OutMax=[]  SumI4OutMin=[]  SumI4OutMax=[]  SumDOutMin=[]  SumDOutMax=[]  DifferentiatorOutMin=[]  DifferentiatorOutMax=[]  FilterDiffOutCoefMin=[]  FilterDiffOutCoefMax=[]  ReciprocalOutMin=[]  ReciprocalOutMax=[]  SumDenOutMin=[]  SumDenOutMax=[]  SumNumOutMin=[]  SumNumOutMax=[]  DivideOutMin=[]  DivideOutMax=[]  UdiffTsProdOutMin=[]  UdiffTsProdOutMax=[]  NTsProdOutMin=[]  NTsProdOutMax=[]  UintegralTsProdOutMin=[]  UintegralTsProdOutMax=[]  UngainTsProdOutMin=[]  UngainTsProdOutMax=[]  IntegratorContinuousStateAttributes=''  IntegratorStateMustResolveToSignalObject=off  IntegratorRTWStateStorageClass=Auto  FilterContinuousStateAttributes=''  FilterStateMustResolveToSignalObject=off  FilterRTWStateStorageClass=Auto  ParallelPVariant=InternalParameters  IdealPVariant=Disabled  IVariant=InternalParameters  DVariant=InternalParameters  IntegratorVariant=Discrete  SatVariant=Disabled  AWVariant=Passthrough  PCopyVariant=Disabled  TRVariant=Disabled  FdbkBlocksVariant=Forward  IdealPFdbkVariant=Disabled  SatFdbkVariant=Disabled  DerivativeFilterVariant=ForwardEulerFilter  NVariant=InternalParameters  NCopyVariant=Disabled  FilterICVariant=InternalICsFilter  IntegratorICVariant=InternalICs  ExternalResetVariant=Disabled  TRSumVariant=Passthrough  SumFdbkVariant=Disabled  SumVariant=Sum_PID  TsampFilterVariant=InternalTs  TsampNgainVariant=Passthrough  TsampIntegralVariant=Passthrough  ExternalSaturationOutDataTypeStr=Inherit: Same as second input
  cfblk5 : ComplexToMagnitudeAngle
  cfblk6 : Product
  cfblk7 : Sum  Inputs=+-
  cfblk8 : MinMax  Inputs=2
  cfblk9 : Gain  Gain=[-895267322.255490]
  cfblk2 : Outport
  cfblk15 : Outport  Port=2
  cfblk16 : Outport  Port=3
  wires:
  cfblk11/1 -> cfblk4/1, cfblk8/2
  cfblk13/1 -> cfblk16/1
  cfblk14/1 -> cfblk7/1, cfblk10/1
  cfblk9/1 -> cfblk3/1
  cfblk10/1 -> cfblk11/1
  cfblk1/1 -> cfblk11/2, cfblk6/2
  cfblk8/1 -> cfblk7/2
  cfblk12/1 -> cfblk5/1
  cfblk3/1 -> cfblk6/1
  cfblk4/1 -> cfblk9/1
  cfblk5/1 -> cfblk3/2
  cfblk7/1 -> cfblk2/1
  cfblk6/1 -> cfblk15/1
  cfblk5/2 -> cfblk8/1

== system sampleModel548_pp_1566_1/cfblk41/cfblk7 ==
  cfblk1 : Inport
  cfblk3 : Sum  Inputs=+-
  cfblk4 : Product  Inputs=*
  cfblk5 : Reshape
  cfblk6 : Constant  Value=[-829717244.065483]  SampleTime=1
  cfblk2 : Outport
  cfblk7 : Outport  Port=2
  cfblk8 : Outport  Port=3
  cfblk9 : Outport  Port=4
  wires:
  cfblk3/1 -> cfblk5/1, cfblk2/1
  cfblk5/1 -> cfblk8/1
  cfblk6/1 -> cfblk4/1, cfblk3/2
  cfblk4/1 -> cfblk9/1, cfblk7/1
  cfblk1/1 -> cfblk3/1

== system sampleModel548_pp_1566_1/cfblk41/cfblk8 ==
  cfblk1 : Inport
  cfblk3 : DiscreteStateSpace
  cfblk4 : DiscreteFilter  SampleTime=1
  cfblk5 : simulink/Discrete/Transfer Fcn Real Zero  ZeroZ=0.75  ICPrevInput=0.0  DoSatur=off
      settings: SourceProductBaseCode=SL
  cfblk6 : Math  Operator=log10  SaturateOnIntegerOverflow=on
  cfblk7 : Signum
  cfblk8 : Constant  Value=[338846521.571194]  SampleTime=1
  cfblk9 : Constant  Value=[-852209918.226592]  SampleTime=1
  cfblk2 : Outport
  cfblk10 : Outport  Port=2
  wires:
  cfblk9/1 -> cfblk2/1
  cfblk5/1 -> cfblk7/1
  cfblk7/1 -> cfblk3/1
  cfblk8/1 -> cfblk6/1
  cfblk1/1 -> cfblk10/1
  cfblk6/1 -> cfblk4/1
  cfblk4/1 -> cfblk5/1

== system sampleModel548_pp_1566_1/cfblk41/cfblk9 ==
  cfblk1 : Inport
  cfblk13 : Inport  Port=2
  cfblk14 : Inport  Port=3
  cfblk10 : Sqrt  Operator=rSqrt  AlgorithmType=Newton-Raphson  SaturateOnIntegerOverflow=on
  cfblk11 : Sin  TimeSource=Use external signal  SampleTime=0
  cfblk12 : Constant  Value=[-247880827.876401]  SampleTime=1
  cfblk17 : Delay  SampleTime=1
  cfblk3 : Trigonometry
  cfblk4 : Product  Inputs=*
  cfblk5 : Product
  cfblk6 : PermuteDimensions
  cfblk7 : Sqrt  SaturateOnIntegerOverflow=on
  cfblk8 : PermuteDimensions
  cfblk9 : Sum  Inputs=|++
  cfblk2 : Outport
  cfblk15 : Outport  Port=2
  cfblk16 : Outport  Port=3
  wires:
  cfblk7/1 -> cfblk5/1
  cfblk1/1 -> cfblk15/1
  cfblk6/1 -> cfblk2/1
  cfblk11/1 -> cfblk7/1
  cfblk9/1 -> cfblk4/1
  cfblk13/1 -> cfblk6/1
  cfblk12/1 -> cfblk16/1
  cfblk14/1 -> cfblk11/1, cfblk8/1
  cfblk5/1 -> cfblk10/1
  cfblk4/1 -> cfblk5/2
  cfblk3/1 -> cfblk9/1
  cfblk8/1 -> cfblk9/2
  cfblk10/1 -> cfblk17/1
  cfblk17/1 -> cfblk3/1

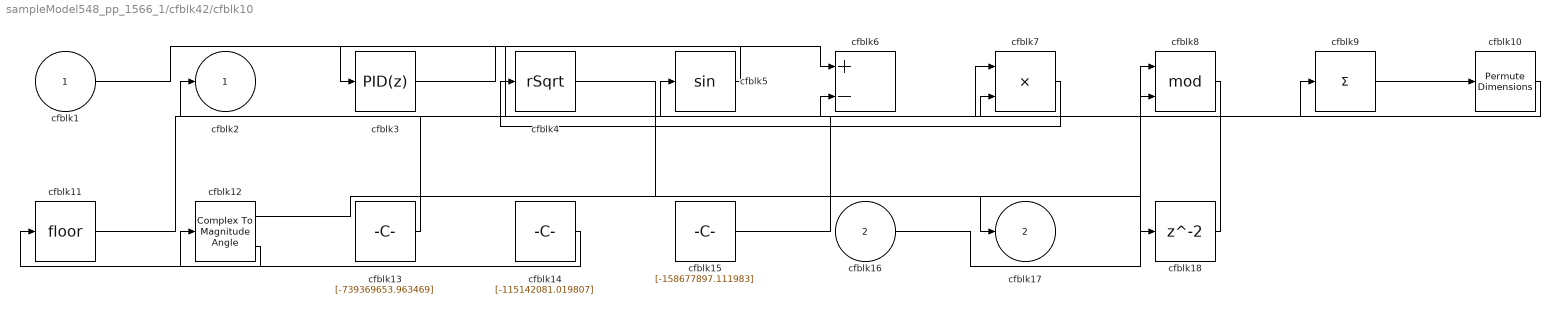
== system sampleModel548_pp_1566_1/cfblk42/cfblk10 ==
  cfblk1 : Inport
  cfblk16 : Inport  Port=2
  cfblk10 : PermuteDimensions
  cfblk11 : Rounding
  cfblk12 : ComplexToMagnitudeAngle
  cfblk13 : Constant  Value=[-739369653.963469]  SampleTime=1
  cfblk14 : Constant  Value=[-115142081.019807]  SampleTime=1
  cfblk15 : Constant  Value=[-158677897.111983]  SampleTime=1
  cfblk18 : Delay  SampleTime=1
  cfblk3 : pid_lib/PID Controller  Controller=PID  Form=Parallel  TimeDomain=Discrete-time  UseExternalTs=off  SampleTime=1  IntegratorMethod=Forward Euler  FilterMethod=Forward Euler  ControllerParametersSource=internal  P=1  I=1  D=0  UseFilter=on  N=100  TunerSelectOption=Transfer Function Based (PID Tuner App)  InitialConditionSource=internal  InitialConditionForIntegrator=0  InitialConditionForFilter=0  DifferentiatorICPrevScaledInput=0  ExternalReset=none  TrackingMode=off  Kt=1  LimitOutput=off  SatLimitsSource=internal  UpperSaturationLimit=inf  LowerSaturationLimit=-inf  LinearizeAsGain=off  AntiWindupMode=none  Kb=1  POutMin=[]  POutMax=[]  IOutMin=[]  IOutMax=[]  DOutMin=[]  DOutMax=[]  NOutMin=[]  NOutMax=[]  SumOutMin=[]  SumOutMax=[]  SaturationOutMin=[]  SaturationOutMax=[]  PParamMin=[]  PParamMax=[]  IParamMin=[]  IParamMax=[]  DParamMin=[]  DParamMax=[]  NParamMin=[]  NParamMax=[]  KbParamMin=[]  KbParamMax=[]  KtParamMin=[]  KtParamMax=[]  KbOutMin=[]  KbOutMax=[]  KtOutMin=[]  KtOutMax=[]  IntegratorOutMin=[]  IntegratorOutMax=[]  FilterOutMin=[]  FilterOutMax=[]  SumI1OutMin=[]  SumI1OutMax=[]  SumI2OutMin=[]  SumI2OutMax=[]  SumI3OutMin=[]  SumI3OutMax=[]  SumI4OutMin=[]  SumI4OutMax=[]  SumDOutMin=[]  SumDOutMax=[]  DifferentiatorOutMin=[]  DifferentiatorOutMax=[]  FilterDiffOutCoefMin=[]  FilterDiffOutCoefMax=[]  ReciprocalOutMin=[]  ReciprocalOutMax=[]  SumDenOutMin=[]  SumDenOutMax=[]  SumNumOutMin=[]  SumNumOutMax=[]  DivideOutMin=[]  DivideOutMax=[]  UdiffTsProdOutMin=[]  UdiffTsProdOutMax=[]  NTsProdOutMin=[]  NTsProdOutMax=[]  UintegralTsProdOutMin=[]  UintegralTsProdOutMax=[]  UngainTsProdOutMin=[]  UngainTsProdOutMax=[]  IntegratorContinuousStateAttributes=''  IntegratorStateMustResolveToSignalObject=off  IntegratorRTWStateStorageClass=Auto  FilterContinuousStateAttributes=''  FilterStateMustResolveToSignalObject=off  FilterRTWStateStorageClass=Auto  ParallelPVariant=InternalParameters  IdealPVariant=Disabled  IVariant=InternalParameters  DVariant=InternalParameters  IntegratorVariant=Discrete  SatVariant=Disabled  AWVariant=Passthrough  PCopyVariant=Disabled  TRVariant=Disabled  FdbkBlocksVariant=Forward  IdealPFdbkVariant=Disabled  SatFdbkVariant=Disabled  DerivativeFilterVariant=ForwardEulerFilter  NVariant=InternalParameters  NCopyVariant=Disabled  FilterICVariant=InternalICsFilter  IntegratorICVariant=InternalICs  ExternalResetVariant=Disabled  TRSumVariant=Passthrough  SumFdbkVariant=Disabled  SumVariant=Sum_PID  TsampFilterVariant=InternalTs  TsampNgainVariant=Passthrough  TsampIntegralVariant=Passthrough  ExternalSaturationOutDataTypeStr=Inherit: Same as second input
  cfblk4 : Sqrt  Operator=rSqrt  AlgorithmType=Newton-Raphson  SaturateOnIntegerOverflow=on
  cfblk5 : Trigonometry
  cfblk6 : Sum  Inputs=+-
  cfblk7 : Product  Inputs=**
  cfblk8 : Math  Operator=mod  SaturateOnIntegerOverflow=on
  cfblk9 : Sum  Inputs=+
  cfblk2 : Outport
  cfblk17 : Outport  Port=2
  wires:
  cfblk12/1 -> cfblk17/1
  cfblk16/1 -> cfblk8/1
  cfblk14/1 -> cfblk12/1
  cfblk12/2 -> cfblk11/1
  cfblk13/1 -> cfblk2/1
  cfblk10/1 -> cfblk8/2
  cfblk1/1 -> cfblk7/2
  cfblk7/1 -> cfblk4/1
  cfblk15/1 -> cfblk9/1
  cfblk9/1 -> cfblk10/1
  cfblk11/1 -> cfblk5/1
  cfblk5/1 -> cfblk3/1
  cfblk3/1 -> cfblk6/1
  cfblk8/1 -> cfblk6/2
  cfblk4/1 -> cfblk18/1
  cfblk18/1 -> cfblk7/1

== system sampleModel548_pp_1566_1/cfblk42/cfblk11 ==
  cfblk1 : Inport
  cfblk12 : Inport  Port=2
  cfblk13 : Inport  Port=3
  cfblk14 : Inport  Port=4
  cfblk15 : Inport  Port=5
  cfblk16 : Inport  Port=6
  cfblk10 : simulink/Math Operations/MinMax Running Resettable  Function=min  vinit=0.0
  cfblk11 : Constant  Value=[-708858344.222618]  SampleTime=1
  cfblk3 : DiscreteStateSpace
  cfblk4 : DiscreteIntegrator  ICPrevOutput=DiscIntNeverNeededParam  ICPrevScaledInput=DiscIntNeverNeededParam
  cfblk5 : UnitDelay  HasFrameUpgradeWarning=on
  cfblk6 : Delay  SampleTime=1
  cfblk7 : Sum  Inputs=-+
  cfblk8 : ComplexToMagnitudeAngle
  cfblk9 : ComplexToRealImag
  cfblk2 : Outport
  wires:
  cfblk15/1 -> cfblk5/1
  cfblk9/1 -> cfblk10/1
  cfblk3/1 -> cfblk7/1
  cfblk13/1 -> cfblk9/1
  cfblk7/1 -> cfblk2/1
  cfblk5/1 -> cfblk10/2
  cfblk6/1 -> cfblk8/1
  cfblk10/1 -> cfblk7/2
  cfblk1/1 -> cfblk6/1
  cfblk9/2 -> cfblk4/1
  cfblk4/1 -> cfblk3/1

== system sampleModel548_pp_1566_1/cfblk42/cfblk8 ==
  cfblk1 : Inport
  cfblk11 : Inport  Port=2
  cfblk12 : Inport  Port=3
  cfblk13 : Inport  Port=4
  cfblk14 : Inport  Port=5
  cfblk10 : Constant  Value=[202416923.947961]  SampleTime=1
  cfblk17 : Delay  SampleTime=1
  cfblk3 : Delay  DelayLengthSource=Input port  SampleTime=1
      settings: InputPortMap=u0,p1
  cfblk4 : simulink/Discrete/Difference  ICPrevInput=0.0  OutMin=[]  OutMax=[]  OutDataTypeStr=Inherit: Inherit via back propagation  OutDataType=fixdt(1, 16)  OutScaling=2^-10  DoSatur=off
  cfblk5 : UnitDelay  HasFrameUpgradeWarning=on
  cfblk6 : MinMax
  cfblk7 : UnaryMinus
  cfblk8 : DotProduct  InputSameDT=on  OutDataTypeStr=Inherit: Inherit via internal rule
  cfblk9 : Constant  Value=[-329113681.085165]  SampleTime=1
  cfblk2 : Outport
  cfblk15 : Outport  Port=2
  cfblk16 : Outport  Port=3
  wires:
  cfblk10/1 -> cfblk5/1
  cfblk4/1 -> cfblk2/1
  cfblk11/1 -> cfblk7/1
  cfblk12/1 -> cfblk15/1
  cfblk13/1 -> cfblk8/1
  cfblk5/1 -> cfblk16/1
  cfblk6/1 -> cfblk8/2
  cfblk9/1 -> cfblk3/1
  cfblk7/1 -> cfblk4/1
  cfblk1/1 -> cfblk3/2
  cfblk8/1 -> cfblk17/1
  cfblk17/1 -> cfblk6/1

== system sampleModel548_pp_1566_1/cfblk42/cfblk9 ==
  cfblk1 : Inport
  cfblk6 : Inport  Port=2
  cfblk7 : Inport  Port=3
  cfblk3 : simulink/Discrete/Transfer Fcn Lead or Lag  PoleZ=0.95  ZeroZ=0.75  ICPrevOutput=0.0  ICPrevInput=0.0  DoSatur=off
      settings: SourceProductBaseCode=SL
  cfblk4 : Delay  DelayLengthSource=Input port  SampleTime=1
      settings: InputPortMap=u0,p1
  cfblk5 : Constant  Value=[-290514364.300051]  SampleTime=1
  cfblk8 : Delay  SampleTime=1
  cfblk2 : Outport
  wires:
  cfblk6/1 -> cfblk2/1
  cfblk7/1 -> cfblk4/1
  cfblk3/1 -> cfblk4/2
  cfblk4/1 -> cfblk8/1
  cfblk8/1 -> cfblk3/1

== system sampleModel548_pp_1566_1/cfblk43/cfblk10 ==
  cfblk1 : Inport
  cfblk7 : Inport  Port=2
  cfblk8 : Inport  Port=3
  cfblk9 : Inport  Port=4
  cfblk10 : Inport  Port=5
  cfblk11 : Inport  Port=6
  cfblk12 : Inport  Port=7
  cfblk13 : Delay  SampleTime=1
  cfblk3 : Polyval  Coefs=[ +2.081618890e-019, -1.441693666e-014, +4.719686976e-010, -8.536869453e-006, +1.621573104e-001, -8.087801117e+001 ]
  cfblk4 : PermuteDimensions
  cfblk5 : ComplexToRealImag
  cfblk6 : Constant  Value=[-161923909.561596]  SampleTime=1
  cfblk2 : Outport
  wires:
  cfblk1/1 -> cfblk2/1
  cfblk3/1 -> cfblk5/1
  cfblk7/1 -> cfblk4/1
  cfblk5/1 -> cfblk13/1
  cfblk13/1 -> cfblk3/1
